simulink model "Test_PIL_IIR_Filter"  (Simulink 8.4)
settings: Solver=FixedStepDiscrete  StartTime=0.0  StopTime=1  FixedStep=0.001  RelTol=1e-3
model workspace (MAT data in the model file):
  dataint = Simulink.Signal
  dataint.DataType = 'int32'
  dataint.Dimensions = -1
  dataint.DimensionsMode = 'auto'
  dataint.Complexity = 'real'
  dataint.SampleTime = -1
  dataint.SamplingMode = 'auto'
  dataint.InitialValue = '0'
PreLoadFcn:
  | run iir_startup;
libraries: simulink x1
settings Model: DataTypeOverrideAppliesTo=Floating-point  Creator=obas  LastModifiedBy=reynaudp
settings DataIOCC: ExternalInput=[t, testdata]  FinalStateName=xFinal_PIL  LimitDataPoints=off  LoadExternalInput=on  SignalLogging=off  StateSaveName=xout_PIL  TimeSaveName=tout_PIL  OutputSaveName=yout_PIL  SignalLoggingName=logsOut_PIL
settings OptimizationCC: ZeroExternalMemoryAtStartup=off  ZeroInternalMemoryAtStartup=off  OptimizeModelRefInitCode=on  LifeSpan=1
settings DebuggingCC: SaveWithParameterizedLinksMsg=none  CheckExecutionContextPreStartOutputMsg=on  CheckExecutionContextRuntimeOutputMsg=on  SignalResolutionControl=TryResolveAllWithWarning  MultiTaskDSMMsg=warning  MultiTaskCondExecSysMsg=none  ParameterPrecisionLossMsg=none  StrictBusMsg=ErrorOnBusTreatedAsVector
settings HardwareCC: ProdLargestAtomicInteger=Integer  ProdLargestAtomicFloat=Float  ProdIntDivRoundTo=Zero  ProdEndianess=LittleEndian  ProdHWDeviceType=STMicroelectronics->STM32 32-bit Cortex-M
settings SFSimCC: SimUserSources=stm32f4xx_rcc
settings RTWCC: SystemTargetFile=stm32.tlc  TemplateMakefile=stm32.tmf  Description=stm32 (Embedded Target)  GenerateReport=on  ProcessScript=stm32_make_rtw_hook  IncludeHyperlinkInReport=on  CodeExecutionProfiling=on  CodeProfilingInstrumentation=on  GenerateCodeReplacementReport=on
settings CodeAppCC: IgnoreCustomStorageClasses=off  MaxIdLength=64  CustomSymbolStrType=$N$R$M  SimulinkBlockComments=off  InternalIdentifier=Classic
settings STFCustomTargetCC: CodeReplacementLibrary=ARM CMSIS SIN COS  ParMdlRefBuildCompliant=on  IncludeMdlTerminateFcn=off  CombineOutputUpdateFcns=on  ERTCustomFileBanners=on  SupportContinuousTime=off  SupportNonInlinedSFcns=off  MATLABClassNameForMDSCustomization=Simulink.SoftwareTarget.ERTCustomization  GRTInterface=off  SystemTargetFile=stm32.tlc
settings ERTTargetCC: CodeReplacementLibrary=ARM CMSIS SIN COS  MultiwordLength=2048  CompOptLevelCompliant=off  ConcurrentExecutionCompliant=off  IncludeMdlTerminateFcn=off  ERTFirstTimeCompliant=off  ModelStepFunctionPrototypeControlCompliant=off  CPPClassGenCompliant=off  InlinedParameterPlacement=NonHierarchical  ERTSrcFileBannerTemplate=sourceFileTemplate.cgt  ERTHdrFileBannerTemplate=sourceFileTemplate.cgt  ERTDataSrcFileTemplate=sourceFileTemplate.cgt  ERTDataHdrFileTemplate=sourceFileTemplate.cgt  ERTCustomFileTemplate=customRoutineProcess.tlc  ConvertIfToSwitch=off  SuppressUnreachableDefaultCases=off
settings CustomProperty: Value=on

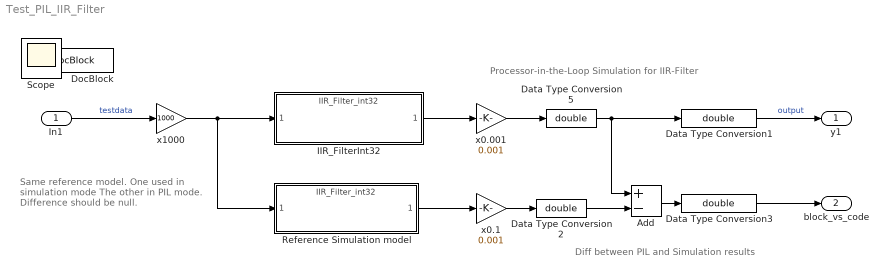
== system Test_PIL_IIR_Filter ==
  note: Same reference model.
      | One used in simulation mode
      | The other in PIL mode.
      | Difference should be null.
  note: Diff between PIL and Simulation results
  note: Processor-in-the-Loop Simulation for IIR-Filter
  In1 : Inport  OutDataTypeStr=double
  Add : Sum  Inputs=+-
  Data Type Conversion{1..3,5} (4 alike) : DataTypeConversion  OutDataTypeStr=double  SaturateOnIntegerOverflow=on  RndMeth=Zero
  DocBlock : simulink/Model-Wide Utilities/DocBlock  DocumentType=Text
      content=|
      | The model contains a 1st-order IIR filter of the following form:
      |
      |     y(n) = a1*y(n-1) + b0*u(n)
      |
      | Using the model pre-load function callback:
      |
      |     a1 = 0.9
      |     b0 = 0.1
      |
      | The filter is sampled at 1000Hz.
      |
      | Modified from iir_filter.mdl to enable ERT code generation.
  IIR_FilterInt32 : ModelReference  ModelNameDialog=IIR_Filter_int32  SimulationMode=Processor-in-the-loop (PIL)  ModelReferenceVersion=1.101  CopyOfModelName=IIR_Filter_int32  DefaultDataLogging=off
  Reference Simulation model : ModelReference  ModelNameDialog=IIR_Filter_int32.mdl  SimulationMode=Normal  ModelReferenceVersion=1.101  CopyOfModelName=IIR_Filter_int32.mdl  DefaultDataLogging=on
  x0.001 : Gain  Gain=0.001
  x0.1 : Gain  Gain=0.001
  x1000 : Gain  Gain=1000  ParamDataTypeStr=uint32  OutMin=-2147483647-1  OutMax=2147483647  OutDataTypeStr=int32
  y1 : Outport
  block_vs_code : Outport  Port=2
  Scope : Scope  NumInputPorts=3
      settings: YMin=-1.5~-1.5~-0.1  YMax=1.5~1.5~0.1  MaxDataPoints=7500
  wires:
  In1/1 -> x1000/1  "testdata"
  Data Type Conversion1/1 -> y1/1  "output"
  Data Type Conversion3/1 -> block_vs_code/1
  Add/1 -> Data Type Conversion3/1
  Data Type Conversion5/1 -> Add/1, Data Type Conversion1/1
  x0.001/1 -> Data Type Conversion5/1
  x1000/1 -> Reference Simulation model/1, IIR_FilterInt32/1
  IIR_FilterInt32/1 -> x0.001/1
  x0.1/1 -> Data Type Conversion2/1
  Reference Simulation model/1 -> x0.1/1
  Data Type Conversion2/1 -> Add/2
